simulink model "Project1_2"  (R2015b)
settings: Solver=ode5  StartTime=0.0  StopTime=5  FixedStep=0.01  RelTol=1e-3
values from neighbouring files (symbols this model uses):
  x0 = 1    [Project1.m]
  x_dot0 = -2    [Project1.m]
settings Model: Creator=Dell  LastModifiedBy=Dell
settings DataIOCC: LimitDataPoints=off

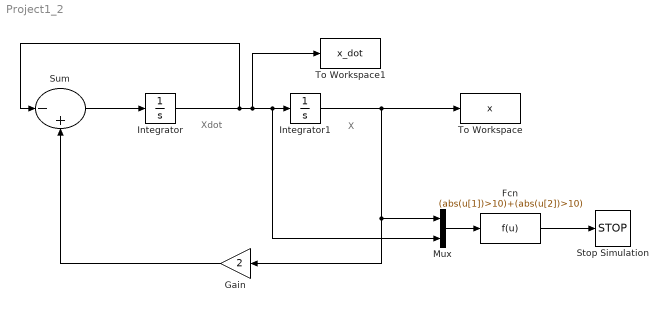
== system Project1_2 ==
  note: X
  note: Xdot
  Fcn : Fcn  Expr=(abs(u[1])>10)+(abs(u[2])>10)
  Gain : Gain  Gain=2
  Integrator : Integrator  InitialCondition=x_dot0
  Integrator1 : Integrator  InitialCondition=x0
  Mux : Mux  Inputs=2
  Stop Simulation : Stop
  Sum : Sum  Inputs=|-+
  To Workspace : ToWorkspace  VariableName=x  SampleTime=-1
  To Workspace1 : ToWorkspace  VariableName=x_dot  SampleTime=-1
  wires:
  Integrator1/1 -> Mux/1, Gain/1, To Workspace/1
  Integrator/1 -> Sum/1, To Workspace1/1, Mux/2, Integrator1/1
  Sum/1 -> Integrator/1
  Gain/1 -> Sum/2
  Mux/1 -> Fcn/1
  Fcn/1 -> Stop Simulation/1
